simulink model "RNN_ConvexOptimization"  (R2020b)
settings: Solver=ode3  StartTime=0.0  StopTime=20  FixedStep=5e-4  RelTol=1e-3
settings Model: Creator=ferna  LastModifiedBy=ferna

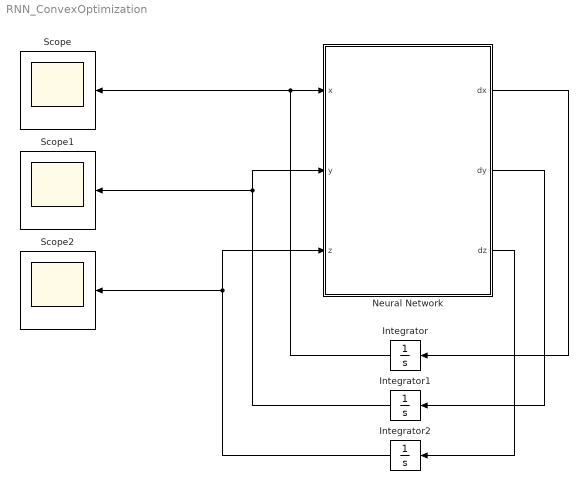
== system RNN_ConvexOptimization ==
  Integrator : Integrator  InitialCondition=[1;-2]
  Integrator1 : Integrator  InitialCondition=1
  Integrator2 : Integrator  InitialCondition=1
  Neural Network : MATLAB Function  TreatAsAtomicUnit=on
  Scope : Scope
  Scope1 : Scope
  Scope2 : Scope
  wires:
  Neural Network/1(dx) -> Integrator/1
  Integrator/1 -> Scope/1, Neural Network/1(x)
  Neural Network/2(dy) -> Integrator1/1
  Integrator1/1 -> Scope1/1, Neural Network/2(y)
  Neural Network/3(dz) -> Integrator2/1
  Integrator2/1 -> Scope2/1, Neural Network/3(z)

== matlab function RNN_ConvexOptimization/Neural Network ==
  data: x input; dx output; y input; z input; dy output; dz output
function [dx,dy,dz] = fcn(x,y,z)
    %%%%%%%%%%%%%%%%%%%%%%%%%
    %% Define The Function %%
    %%%%%%%%%%%%%%%%%%%%%%%%%
    % f = (x(1)-2)^2 + (x(2)-1)^2;
    
    %%%%%%%%%%%%%%%%%%%%%%%%%
    %% Partial Derivatives %%
    %%%%%%%%%%%%%%%%%%%%%%%%%
    dfx1 = 2*x(1) - 4;     % eval(diff(f,x1));
    dfx2 = 2*x(2) - 2;     % eval(diff(f,x2));
    dfx = [dfx1;dfx2];
    
    %%%%%%%%%%%%%%%%%%%%%%%%
    %% Define Constraints %%
    %%%%%%%%%%%%%%%%%%%%%%%%
    % Inequality Constraints %
    gx = 0.25*(x(1)^2) + x(2)^2 - 1;
    dgx1 = x(1)/2;          % diff(gx,x1);
    dgx2 = 2*x(2);          %diff(gx,x2);
    
    dgx = [dgx1;dgx2];
    
    % Equality Constraints %
    % h = x1 - 2*x2 = -1
    A = [1,-2];
    b = -1;
    
    %%%%%%%%%%%%%%%%%%%%%%%%%%%%%%
    %% Define Bound Constraints %%
    %%%%%%%%%%%%%%%%%%%%%%%%%%%%%%
    % Upper Bound %
    LowB = [-3;-3]; 
    % Upper bound %
    UpB = [3;3]; 

    %%%%%%%%%%%%%%%%%%%%%%%%%%%
    %% Apply the Projections %%
    %%%%%%%%%%%%%%%%%%%%%%%%%%%
    xi = x - dfx - dgx*y + A'*z;
    
    Px = zeros(length(xi),1);
    for n=1:length(xi)
        Px(n,1) = piecewisex(LowB(n),UpB(n),xi(n)); 
    end
    
    %%%%%%%%%%%%%%%%%%%%%%%%%%%%%%%
    %% Neural Network Structures %%
    %%%%%%%%%%%%%%%%%%%%%%%%%%%%%%%
    dx = -x + Px;
    dy = -y + max(y + gx,0);
    dz = -A*x + b;
    
end 

%%%%%%%%%%%%%%%%%%%%%%%%%%%%%%%%%%%%
% Evaluation of PieceWise Function %
%%%%%%%%%%%%%%%%%%%%%%%%%%%%%%%%%%%%
% Piecewise Function For States x1, x2, x3 & x4 %
function y = piecewisex(Lbx, Ubx, xin)
    y = 0;
    idx1 = xin <= Lbx;
    y(idx1) = Lbx;
    idx2 = xin >= Ubx;
    y(idx2) = Ubx;
    y(~(idx1 | idx2)) = xin;
end
